simulink model "StopwatchSpec"  (R2017b)
settings: Solver=FixedStepDiscrete  StartTime=0.0  StopTime=20  FixedStep=1  RelTol=1e-3
model workspace (MAT data in the model file):
  ContractValidatorBlocksMap = containers.Map
  ContractValidatorBlocksMap.serialization.keys = {'StopwatchSpec/contract/validator'}
  ContractValidatorBlocksMap.serialization.values{1}.block = 'StopwatchSpec/contract/validator'
  ContractValidatorBlocksMap.serialization.values{1}.assumePorts = 1
  ContractValidatorBlocksMap.serialization.values{1}.guaranteePorts = 3
  ContractValidatorBlocksMap.serialization.values{1}.modeBlocksPorts = 3
  ContractValidatorBlocksMap.serialization.values{1}.portHandles.Inport = [348.002807617 349.003417969 350.003173828 351.002075195 352.002319336 353.002319336 354.004394531]
  ContractValidatorBlocksMap.serialization.values{1}.portHandles.Outport = 355.00402832
  ContractValidatorBlocksMap.serialization.values{1}.portHandles.Enable = []
  ContractValidatorBlocksMap.serialization.values{1}.portHandles.Trigger = []
  ContractValidatorBlocksMap.serialization.values{1}.portHandles.State = []
  ContractValidatorBlocksMap.serialization.values{1}.portHandles.LConn = []
  ContractValidatorBlocksMap.serialization.values{1}.portHandles.RConn = []
  ContractValidatorBlocksMap.serialization.values{1}.portHandles.Ifaction = []
  ContractValidatorBlocksMap.serialization.values{1}.portHandles.Reset = []
  ContractValidatorBlocksMap.serialization.values{1}.portConnectivity(1).Type = '1'
  ContractValidatorBlocksMap.serialization.values{1}.portConnectivity(1).Position = [490 -60]
  ContractValidatorBlocksMap.serialization.values{1}.portConnectivity(1).SrcBlock = 14.0024414062
  ContractValidatorBlocksMap.serialization.values{1}.portConnectivity(1).SrcPort = 0
  ContractValidatorBlocksMap.serialization.values{1}.portConnectivity(1).DstBlock = []
  ContractValidatorBlocksMap.serialization.values{1}.portConnectivity(1).DstPort = []
  ContractValidatorBlocksMap.serialization.values{1}.portConnectivity(2).Type = '2'
  ContractValidatorBlocksMap.serialization.values{1}.portConnectivity(2).Position = [490 35]
  ContractValidatorBlocksMap.serialization.values{1}.portConnectivity(2).SrcBlock = 117.002685547
  ContractValidatorBlocksMap.serialization.values{1}.portConnectivity(2).SrcPort = 0
  ContractValidatorBlocksMap.serialization.values{1}.portConnectivity(2).DstBlock = []
  ContractValidatorBlocksMap.serialization.values{1}.portConnectivity(2).DstPort = []
  ContractValidatorBlocksMap.serialization.values{1}.portConnectivity(3).Type = '3'
  ContractValidatorBlocksMap.serialization.values{1}.portConnectivity(3).Position = [490 130]
  ContractValidatorBlocksMap.serialization.values{1}.portConnectivity(3).SrcBlock = 84.0024414062
  ContractValidatorBlocksMap.serialization.values{1}.portConnectivity(3).SrcPort = 0
  ContractValidatorBlocksMap.serialization.values{1}.portConnectivity(3).DstBlock = []
  ContractValidatorBlocksMap.serialization.values{1}.portConnectivity(3).DstPort = []
  ContractValidatorBlocksMap.serialization.values{1}.portConnectivity(4).Type = '4'
  ContractValidatorBlocksMap.serialization.values{1}.portConnectivity(4).Position = [490 225]
  ContractValidatorBlocksMap.serialization.values{1}.portConnectivity(4).SrcBlock = 111.003662109
  ContractValidatorBlocksMap.serialization.values{1}.portConnectivity(4).SrcPort = 0
  ContractValidatorBlocksMap.serialization.values{1}.portConnectivity(4).DstBlock = []
  ContractValidatorBlocksMap.serialization.values{1}.portConnectivity(4).DstPort = []
  ContractValidatorBlocksMap.serialization.values{1}.portConnectivity(5).Type = '5'
  ContractValidatorBlocksMap.serialization.values{1}.portConnectivity(5).Position = [490 320]
  ContractValidatorBlocksMap.serialization.values{1}.portConnectivity(5).SrcBlock = 175.004272461
  ContractValidatorBlocksMap.serialization.values{1}.portConnectivity(5).SrcPort = 0
  ContractValidatorBlocksMap.serialization.values{1}.portConnectivity(5).DstBlock = []
  ContractValidatorBlocksMap.serialization.values{1}.portConnectivity(5).DstPort = []
  ContractValidatorBlocksMap.serialization.values{1}.portConnectivity(6).Type = '6'
  ContractValidatorBlocksMap.serialization.values{1}.portConnectivity(6).Position = [490 415]
  ContractValidatorBlocksMap.serialization.values{1}.portConnectivity(6).SrcBlock = 186.00378418
  ContractValidatorBlocksMap.serialization.values{1}.portConnectivity(6).SrcPort = 0
  ContractValidatorBlocksMap.serialization.values{1}.portConnectivity(6).DstBlock = []
  ContractValidatorBlocksMap.serialization.values{1}.portConnectivity(6).DstPort = []
  ContractValidatorBlocksMap.serialization.values{1}.portConnectivity(7).Type = '7'
  ContractValidatorBlocksMap.serialization.values{1}.portConnectivity(7).Position = [490 510]
  ContractValidatorBlocksMap.serialization.values{1}.portConnectivity(7).SrcBlock = 197.002929688
  ContractValidatorBlocksMap.serialization.values{1}.portConnectivity(7).SrcPort = 0
  ContractValidatorBlocksMap.serialization.values{1}.portConnectivity(7).DstBlock = []
  ContractValidatorBlocksMap.serialization.values{1}.portConnectivity(7).DstPort = []
  ContractValidatorBlocksMap.serialization.values{1}.portConnectivity(8).Type = '1'
  ContractValidatorBlocksMap.serialization.values{1}.portConnectivity(8).Position = [595 225]
  ContractValidatorBlocksMap.serialization.values{1}.portConnectivity(8).SrcBlock = []
  ContractValidatorBlocksMap.serialization.values{1}.portConnectivity(8).SrcPort = []
  ContractValidatorBlocksMap.serialization.values{1}.portConnectivity(8).DstBlock = 209.004150391
  ContractValidatorBlocksMap.serialization.values{1}.portConnectivity(8).DstPort = 0
  ContractValidatorBlocksMap.serialization.uniformity = 0
  ContractValidatorBlocksMap.serialization.keyType = 'char'
  ContractValidatorBlocksMap.serialization.valueType = 'any'
undefined symbols (not defined in the file or in its folder): ArrowOperator, contractAfterSimulation, ContractAssumeBlock, contractBeforeSimulation, ContractBlock, ContractEnsureBlock, ContractGuaranteeBlock, ContractModeBlock, ContractRequireBlock, ContractValidatorBlock, saveValidatorParameters
libraries: simulink x7, Kind x1
settings Model: Creator=mahgoubyahia  LastModifiedBy=hbourbou
settings OptimizationCC: LifeSpan=inf
settings DebuggingCC: SFExecutionAtInitializationDiag=none
settings HardwareCC: ProdBitPerSizeT=32  ProdBitPerPtrDiffT=32  ProdWordSize=32  ProdHWDeviceType=Specified
settings CodeAppCC: StateflowObjectComments=on

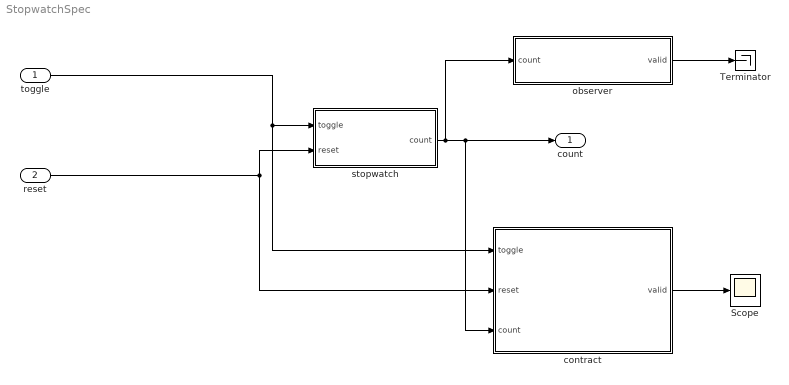
== system StopwatchSpec ==
  toggle : Inport
  reset : Inport  Port=2
  Scope : Scope
  Terminator : Terminator
  contract : Subsystem  AncestorBlock=Kind/contract  mask(ContractBlock){ContractBlockType=ContractBlock}
      mask DialogControl DescTextVar Prompt: Contract block
      mask Display:
      | text(0.5, 0.5, '{\bf\fontsize{20}Contract}', 'hor', 'center', 'texmode','on');
      | blocks = find_system(gcb, 'LookUnderMasks','all', 'SearchDepth',1,'BlockType','Inport');
      | for i = 1 : length(blocks)
      |     blockName = get_param(blocks(i), 'Name');
      |     [path, blockName] = fileparts(char(blockName));
      |     port_label('input', i, blockName);
      | end
      | 
      | blocks = find_system(gcb, 'LookUnderMasks','all', 'SearchDepth',1,'BlockType','Outport');
      | for i = 1 : length(blocks)
      |     blockName = get_param(blocks(i), 'Name');
      |     [path, blockName] = fileparts(char(blockName));
      |     port_label('output', i, blockName);
      | end
  observer : Subsystem  TreatAsAtomicUnit=on  mask(Observer){AnnotationType=ensures, ObserverType=ellipsoid}
      mask prompts: AnnotationType "Type of annotation (pre/post...)"; ObserverType "Observer type"
      mask help:
      | Set an observer for the system.
      | The annotation type parameter sets the type of observer:
      | - requires : pre-condition
      | - ensures : post-condition
      | - assert : an assertion
      | - observer : the observer computes a special type of properties
      mask TypeOptions AnnotationType: ensures | requires | assert | observer
      mask Callback AnnotationType:
      | paramStr = get_param(gcb, 'MaskValues');
      | 
      | if strcmp(paramStr{1}(1),'o')
      |     set_param(gcb,'MaskVisibilities',{'on';'on'});
      |     paramStr{2} = 'ellipsoid';
      |     set_param(gcb,'MaskValues',paramStr);
      | else
      |     set_param(gcb,'MaskVisibilities',{'on';'off'});
      | end
      mask Callback ObserverType:
      | paramStr = get_param(gcb, 'MaskValues');
      | 
      | if strcmp(paramStr{1}(1),'observer')
      |     set_param(gcb,'MaskVisibilities',{'on';'on'});
      |     paramStr{2} = 'ellipsoid';
      |     set_param(gcb,'MaskValues',paramStr);
      | else
      |     set_param(gcb,'MaskVisibilities',{'on';'off'});
      | end
      mask Display:
      | color('black');
      | text(0.5, 0.5, 'Observer Block', 'horizontalAlignment', 'center');
  stopwatch : Subsystem
  count : Outport
  wires:
  contract/1(valid) -> Scope/1
  reset/1 -> stopwatch/2(reset), contract/2(reset)
  toggle/1 -> contract/1(toggle), stopwatch/1(toggle)
  observer/1(valid) -> Terminator/1
  stopwatch/1(count) -> count/1, contract/3(count), observer/1(count)

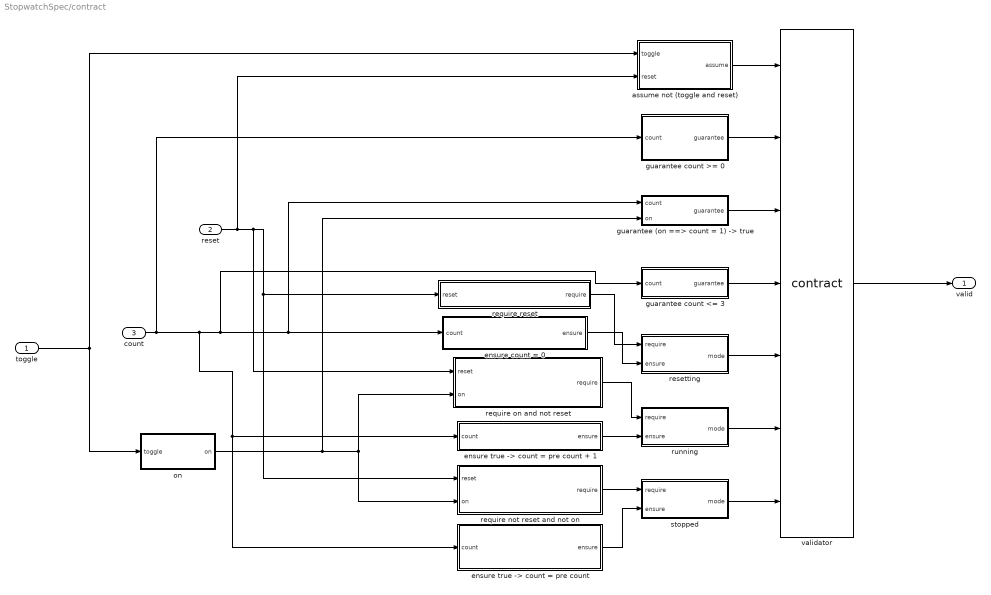
== system StopwatchSpec/contract ==
  toggle : Inport
  reset : Inport  Port=2
  count : Inport  Port=3  OutDataTypeStr=int32
  assume not (toggle and reset) : Subsystem  AncestorBlock=Kind/assume  mask(ContractAssumeBlock){ContractBlockType=ContractAssumeBlock}
      mask DialogControl DescTextVar Prompt: Assume block
  ensure count = 0 : Subsystem  AncestorBlock=Kind/ensure  mask(ContractEnsureBlock){ContractBlockType=ContractEnsureBlock}
      mask DialogControl DescTextVar Prompt: Ensure block
  "ensure true -> count = pre count" : Subsystem  AncestorBlock=Kind/ensure  mask(ContractEnsureBlock){ContractBlockType=ContractEnsureBlock}
      mask DialogControl DescTextVar Prompt: Ensure block
  "ensure true -> count = pre count + 1" : Subsystem  AncestorBlock=Kind/ensure  mask(ContractEnsureBlock){ContractBlockType=ContractEnsureBlock}
      mask DialogControl DescTextVar Prompt: Ensure block
  "guarantee (on ==> count = 1) -> true " : Subsystem  mask(ContractGuaranteeBlock){ContractBlockType=ContractGuaranteeBlock}
      mask DialogControl DescTextVar Prompt: Guarantee block
  guarantee count <= 3 : Subsystem  mask(ContractGuaranteeBlock){ContractBlockType=ContractGuaranteeBlock}
      mask DialogControl DescTextVar Prompt: Guarantee block
  guarantee count >= 0 : Subsystem  AncestorBlock=Kind/guarantee  mask(ContractGuaranteeBlock){ContractBlockType=ContractGuaranteeBlock}
      mask DialogControl DescTextVar Prompt: Guarantee block
  on : Subsystem
  require not reset and not on : Subsystem  AncestorBlock=Kind/require  mask(ContractRequireBlock){ContractBlockType=ContractRequireBlock}
      mask DialogControl DescTextVar Prompt: Require block
  require on and not reset : Subsystem  AncestorBlock=Kind/require  mask(ContractRequireBlock){ContractBlockType=ContractRequireBlock}
      mask DialogControl DescTextVar Prompt: Require block
  require reset : Subsystem  AncestorBlock=Kind/require  mask(ContractRequireBlock){ContractBlockType=ContractRequireBlock}
      mask DialogControl DescTextVar Prompt: Require block
  resetting : Subsystem  AncestorBlock=Kind/mode  mask(ContractModeBlock){ContractBlockType=ContractModeBlock}
      mask DialogControl DescTextVar Prompt: Mode block
  running : Subsystem  AncestorBlock=Kind/mode  mask(ContractModeBlock){ContractBlockType=ContractModeBlock}
      mask DialogControl DescTextVar Prompt: Mode block
  stopped : Subsystem  AncestorBlock=Kind/mode  mask(ContractModeBlock){ContractBlockType=ContractModeBlock}
      mask DialogControl DescTextVar Prompt: Mode block
  validator : M-S-Function  LoadFcn=saveValidatorParameters(gcb);  InitFcn=contractBeforeSimulation();  StopFcn=contractAfterSimulation();  FunctionName=contract  mask(ContractValidatorBlock){assumePorts=1, guaranteePorts=3, modePorts=3, ContractBlockType=ContractValidatorBlock, createInportsCheckbox=off}
      mask prompts: assumePorts "Assume ports     :"; guaranteePorts "Guarantee ports :"; modePorts "Mode ports        :"; createInportsCheckbox "Create inports and connect them automatically"
      mask init:
      | set_param(gcb,'LinkStatus','none');
      | contract_callback('inputs_callback',gcb);
      mask DialogControl DescTextVar Prompt: The validator block implements the following logic: <br> <br> <b>Sofar</b>(assume<sub>1</sub> <b>&#8743;</b> assume<sub>2</sub> <b>&#8743;</b> ... assume<sub>k</sub>) <b>&rarr;</b> (guarantee<sub>1</sub> <b>&#8743;</b> guarantee<sub>2</sub> <b>&#8743;</b> ... guarantee<sub>m</sub> <b>&#8743;</b>  mode<sub>1</sub> <b>&#8743;</b> mode<sub>2</sub> <b>&#8743;</b> ... <b>&#8743;</b> mode<sub>n</sub> )<br> where mode<sub>i</sub> = require<sub>i</sub> <b>&rarr;</b> ensure<sub>i</sub>
      mask Display:
      | color('black');
      | port_label('input',1,'assume');
      | port_label('input',2,'guarantee');
      | port_label('input',3,'guarantee');
      | port_label('input',4,'guarantee');
      | port_label('input',5,'mode');
      | port_label('input',6,'mode');
      | port_label('input',7,'mode');
      | port_label('output',1,'valid');
  valid : Outport
  wires:
  toggle/1 -> on/1(toggle), assume not (toggle and reset)/1(toggle)
  reset/1 -> require on and not reset/1(reset), require reset/1(reset), require not reset and not on/1(reset), assume not (toggle and reset)/2(reset)
  ensure count = 0/1(ensure) -> resetting/2(ensure)
  require on and not reset/1(require) -> running/1(require)
  "ensure true -> count = pre count + 1"/1(ensure) -> running/2(ensure)
  require not reset and not on/1(require) -> stopped/1(require)
  "ensure true -> count = pre count"/1(ensure) -> stopped/2(ensure)
  on/1(on) -> "guarantee (on ==> count = 1) -> true "/2(on), require on and not reset/2(on), require not reset and not on/2(on)
  count/1 -> guarantee count >= 0/1(count), "ensure true -> count = pre count"/1(count), "ensure true -> count = pre count + 1"/1(count), guarantee count <= 3/1(count), "guarantee (on ==> count = 1) -> true "/1(count), ensure count = 0/1(count)
  require reset/1(require) -> resetting/1(require)
  validator/1 -> valid/1
  assume not (toggle and reset)/1(assume) -> validator/1
  guarantee count >= 0/1(guarantee) -> validator/2
  "guarantee (on ==> count = 1) -> true "/1(guarantee) -> validator/3
  resetting/1(mode) -> validator/5
  running/1(mode) -> validator/6
  stopped/1(mode) -> validator/7
  guarantee count <= 3/1(guarantee) -> validator/4

== system StopwatchSpec/observer ==
  count : Inport
  Compare To Constant : simulink/Logic and Bit Operations/Compare To Constant  relop=<=  const=2  OutDataTypeStr=boolean
  valid : Outport
  wires:
  Compare To Constant/1 -> valid/1
  count/1 -> Compare To Constant/1

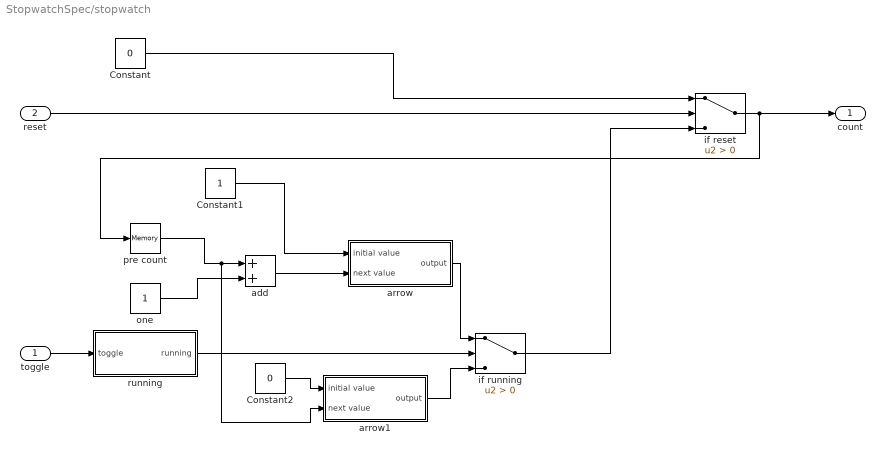
== system StopwatchSpec/stopwatch ==
  toggle : Inport
  reset : Inport  Port=2
  Constant : Constant  Value=0  OutDataTypeStr=int32
  Constant1 : Constant  OutDataTypeStr=int32
  Constant2 : Constant  Value=0  OutDataTypeStr=int32
  add : Sum
  arrow : Subsystem  mask{LustreOperatorBlock=ArrowOperator}
      mask prompts: LustreOperatorBlock "ArrowOperator"
  arrow1 : Subsystem  mask{LustreOperatorBlock=ArrowOperator}
      mask prompts: LustreOperatorBlock "ArrowOperator"
  if reset : Switch  Criteria=u2 > Threshold
  if running : Switch  Criteria=u2 > Threshold
  one : Constant  OutDataTypeStr=int32
  pre count : Memory
  running : Subsystem
  count : Outport
  wires:
  running/1(running) -> if running/2
  if reset/1 -> count/1, pre count/1
  if running/1 -> if reset/3
  reset/1 -> if reset/2
  Constant/1 -> if reset/1
  one/1 -> add/2
  toggle/1 -> running/1(toggle)
  Constant1/1 -> arrow/1(initial value)
  add/1 -> arrow/2(next value)
  arrow/1(output) -> if running/1
  pre count/1 -> arrow1/2(next value), add/1
  Constant2/1 -> arrow1/1(initial value)
  arrow1/1(output) -> if running/3

== system StopwatchSpec/contract/assume not (toggle and reset) ==
  toggle : Inport
  reset : Inport  Port=2
  and : Logic  IconShape=distinctive  AllPortsSameDT=off  OutDataTypeStr=boolean
  not : Logic  Operator=NOT  IconShape=distinctive  AllPortsSameDT=off  OutDataTypeStr=boolean
  assume : Outport  OutDataTypeStr=boolean
  wires:
  toggle/1 -> and/1
  reset/1 -> and/2
  and/1 -> not/1
  not/1 -> assume/1

== system StopwatchSpec/contract/ensure count = 0 ==
  count : Inport
  Compare To Zero : simulink/Logic and Bit Operations/Compare To Zero  relop===  OutDataTypeStr=boolean
  ensure : Outport  OutDataTypeStr=boolean
  wires:
  count/1 -> Compare To Zero/1
  Compare To Zero/1 -> ensure/1

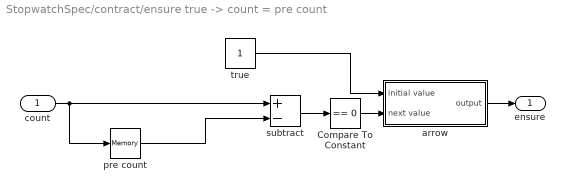
== system StopwatchSpec/contract/ensure true -> count = pre count ==
  count : Inport
  Compare To Constant : simulink/Logic and Bit Operations/Compare To Constant  relop===  const=0  OutDataTypeStr=boolean
  arrow : Subsystem  mask{LustreOperatorBlock=ArrowOperator}
      mask prompts: LustreOperatorBlock "ArrowOperator"
  pre count : Memory
  subtract : Sum  Inputs=+-
  true : Constant  OutDataTypeStr=boolean
  ensure : Outport  OutDataTypeStr=boolean
  wires:
  arrow/1(output) -> ensure/1
  pre count/1 -> subtract/2
  Compare To Constant/1 -> arrow/2(next value)
  count/1 -> pre count/1, subtract/1
  subtract/1 -> Compare To Constant/1
  true/1 -> arrow/1(initial value)

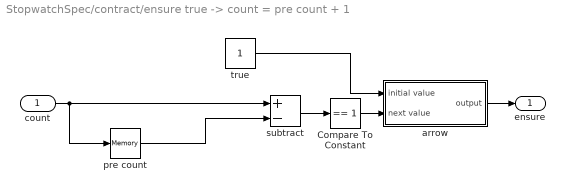
== system StopwatchSpec/contract/ensure true -> count = pre count + 1 ==
  count : Inport
  Compare To Constant : simulink/Logic and Bit Operations/Compare To Constant  relop===  const=1  OutDataTypeStr=boolean
  arrow : Subsystem  mask{LustreOperatorBlock=ArrowOperator}
      mask prompts: LustreOperatorBlock "ArrowOperator"
  pre count : Memory
  subtract : Sum  Inputs=+-
  true : Constant  OutDataTypeStr=boolean
  ensure : Outport  OutDataTypeStr=boolean
  wires:
  count/1 -> pre count/1, subtract/1
  subtract/1 -> Compare To Constant/1
  Compare To Constant/1 -> arrow/2(next value)
  true/1 -> arrow/1(initial value)
  arrow/1(output) -> ensure/1
  pre count/1 -> subtract/2

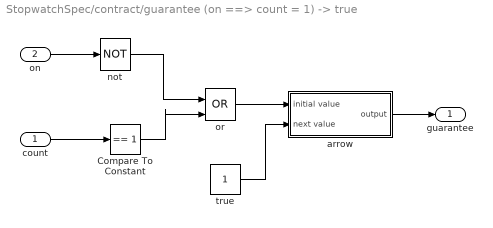
== system StopwatchSpec/contract/guarantee (on ==> count = 1) -> true  ==
  count : Inport  OutDataTypeStr=int32
  on : Inport  Port=2  OutDataTypeStr=boolean
  Compare To Constant : simulink/Logic and Bit Operations/Compare To Constant  relop===  const=1  OutDataTypeStr=boolean
  arrow : Subsystem  mask{LustreOperatorBlock=ArrowOperator}
      mask prompts: LustreOperatorBlock "ArrowOperator"
  not : Logic  Operator=NOT  IconShape=distinctive  AllPortsSameDT=off  OutDataTypeStr=boolean
  or : Logic  Operator=OR  IconShape=distinctive  AllPortsSameDT=off  OutDataTypeStr=boolean
  true : Constant  OutDataTypeStr=boolean
  guarantee : Outport  OutDataTypeStr=boolean
  wires:
  count/1 -> Compare To Constant/1
  Compare To Constant/1 -> or/2
  on/1 -> not/1
  not/1 -> or/1
  or/1 -> arrow/1(initial value)
  true/1 -> arrow/2(next value)
  arrow/1(output) -> guarantee/1

== system StopwatchSpec/contract/guarantee count <= 3 ==
  count : Inport
  Compare To Constant : simulink/Logic and Bit Operations/Compare To Constant  relop=<=  const=3.0  OutDataTypeStr=boolean
  guarantee : Outport  OutDataTypeStr=boolean
  wires:
  count/1 -> Compare To Constant/1
  Compare To Constant/1 -> guarantee/1

== system StopwatchSpec/contract/guarantee count >= 0 ==
  count : Inport
  Compare To Zero : simulink/Logic and Bit Operations/Compare To Zero  relop=>=  OutDataTypeStr=boolean
  guarantee : Outport  OutDataTypeStr=boolean
  wires:
  count/1 -> Compare To Zero/1
  Compare To Zero/1 -> guarantee/1

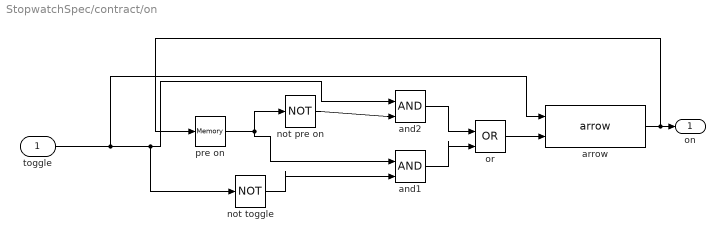
== system StopwatchSpec/contract/on ==
  toggle : Inport
  and1 : Logic  IconShape=distinctive  AllPortsSameDT=off  OutDataTypeStr=boolean
  and2 : Logic  IconShape=distinctive  AllPortsSameDT=off  OutDataTypeStr=boolean
  arrow : Kind/arrow  LustreOperatorBlock=ArrowOperator
  not pre on : Logic  Operator=NOT  IconShape=distinctive  AllPortsSameDT=off  OutDataTypeStr=boolean
  not toggle : Logic  Operator=NOT  IconShape=distinctive  AllPortsSameDT=off  OutDataTypeStr=boolean
  or : Logic  Operator=OR  IconShape=distinctive  AllPortsSameDT=off  OutDataTypeStr=boolean
  pre on : Memory
  on : Outport
  wires:
  toggle/1 -> arrow/1, not toggle/1, and2/1
  not toggle/1 -> and1/2
  pre on/1 -> and1/1, not pre on/1
  not pre on/1 -> and2/2
  and2/1 -> or/1
  and1/1 -> or/2
  or/1 -> arrow/2
  arrow/1 -> pre on/1, on/1

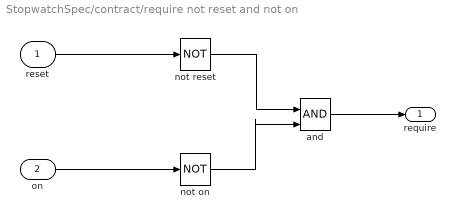
== system StopwatchSpec/contract/require not reset and not on ==
  reset : Inport
  on : Inport  Port=2
  and : Logic  IconShape=distinctive  AllPortsSameDT=off  OutDataTypeStr=boolean
  not on : Logic  Operator=NOT  IconShape=distinctive  AllPortsSameDT=off  OutDataTypeStr=boolean
  not reset : Logic  Operator=NOT  IconShape=distinctive  AllPortsSameDT=off  OutDataTypeStr=boolean
  require : Outport  OutDataTypeStr=boolean
  wires:
  reset/1 -> not reset/1
  on/1 -> not on/1
  not reset/1 -> and/1
  not on/1 -> and/2
  and/1 -> require/1

== system StopwatchSpec/contract/require on and not reset ==
  reset : Inport
  on : Inport  Port=2
  and : Logic  IconShape=distinctive  AllPortsSameDT=off  OutDataTypeStr=boolean
  not reset : Logic  Operator=NOT  IconShape=distinctive  AllPortsSameDT=off  OutDataTypeStr=boolean
  require : Outport  OutDataTypeStr=boolean
  wires:
  on/1 -> and/2
  reset/1 -> not reset/1
  not reset/1 -> and/1
  and/1 -> require/1

== system StopwatchSpec/contract/require reset ==
  reset : Inport
  require : Outport  OutDataTypeStr=boolean
  wires:
  reset/1 -> require/1

== system StopwatchSpec/contract/resetting ==
  note: Shouldn't not be edited
  require : Inport  OutDataTypeStr=boolean
  ensure : Inport  Port=2  OutDataTypeStr=boolean
  and : Logic  Operator=NOT  IconShape=distinctive  AllPortsSameDT=off  OutDataTypeStr=boolean
  or : Logic  Operator=OR  IconShape=distinctive  AllPortsSameDT=off  OutDataTypeStr=boolean
  mode : Outport
  wires:
  require/1 -> and/1
  ensure/1 -> or/2
  and/1 -> or/1
  or/1 -> mode/1

== system StopwatchSpec/contract/running ==
  note: Shouldn't not be edited
  require : Inport  OutDataTypeStr=boolean
  ensure : Inport  Port=2  OutDataTypeStr=boolean
  and : Logic  Operator=NOT  IconShape=distinctive  AllPortsSameDT=off  OutDataTypeStr=boolean
  or : Logic  Operator=OR  IconShape=distinctive  AllPortsSameDT=off  OutDataTypeStr=boolean
  mode : Outport
  wires:
  require/1 -> and/1
  ensure/1 -> or/2
  and/1 -> or/1
  or/1 -> mode/1

== system StopwatchSpec/contract/stopped ==
  note: Shouldn't not be edited
  require : Inport  OutDataTypeStr=boolean
  ensure : Inport  Port=2  OutDataTypeStr=boolean
  and : Logic  Operator=NOT  IconShape=distinctive  AllPortsSameDT=off  OutDataTypeStr=boolean
  or : Logic  Operator=OR  IconShape=distinctive  AllPortsSameDT=off  OutDataTypeStr=boolean
  mode : Outport
  wires:
  require/1 -> and/1
  ensure/1 -> or/2
  and/1 -> or/1
  or/1 -> mode/1

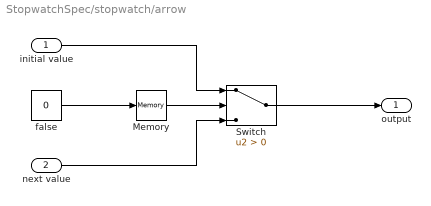
== system StopwatchSpec/stopwatch/arrow ==
  initial value : Inport
  next value : Inport  Port=2
  Memory : Memory  InitialCondition=1
  Switch : Switch  Criteria=u2 > Threshold
  false : Constant  Value=0  OutDataTypeStr=boolean
  output : Outport
  wires:
  Switch/1 -> output/1
  next value/1 -> Switch/3
  Memory/1 -> Switch/2
  false/1 -> Memory/1
  initial value/1 -> Switch/1

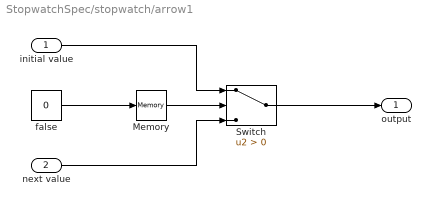
== system StopwatchSpec/stopwatch/arrow1 ==
  initial value : Inport
  next value : Inport  Port=2
  Memory : Memory  InitialCondition=1
  Switch : Switch  Criteria=u2 > Threshold
  false : Constant  Value=0  OutDataTypeStr=boolean
  output : Outport
  wires:
  Switch/1 -> output/1
  next value/1 -> Switch/3
  Memory/1 -> Switch/2
  false/1 -> Memory/1
  initial value/1 -> Switch/1

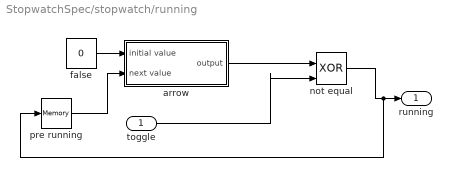
== system StopwatchSpec/stopwatch/running ==
  toggle : Inport
  arrow : Subsystem  mask{LustreOperatorBlock=ArrowOperator}
      mask prompts: LustreOperatorBlock "ArrowOperator"
  false : Constant  Value=0  OutDataTypeStr=boolean
  not equal : Logic  Operator=XOR  IconShape=distinctive  AllPortsSameDT=off  OutDataTypeStr=boolean
  pre running : Memory
  running : Outport
  wires:
  false/1 -> arrow/1(initial value)
  arrow/1(output) -> not equal/1
  not equal/1 -> pre running/1, running/1
  toggle/1 -> not equal/2
  pre running/1 -> arrow/2(next value)

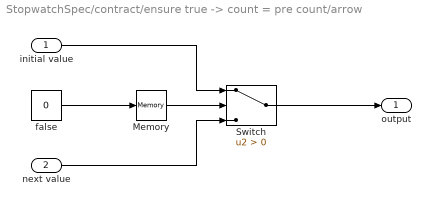
== system StopwatchSpec/contract/ensure true -> count = pre count/arrow ==
  initial value : Inport
  next value : Inport  Port=2
  Memory : Memory  InitialCondition=1
  Switch : Switch  Criteria=u2 > Threshold
  false : Constant  Value=0  OutDataTypeStr=boolean
  output : Outport
  wires:
  Switch/1 -> output/1
  next value/1 -> Switch/3
  Memory/1 -> Switch/2
  false/1 -> Memory/1
  initial value/1 -> Switch/1

== system StopwatchSpec/contract/ensure true -> count = pre count + 1/arrow ==
  initial value : Inport
  next value : Inport  Port=2
  Memory : Memory  InitialCondition=1
  Switch : Switch  Criteria=u2 > Threshold
  false : Constant  Value=0  OutDataTypeStr=boolean
  output : Outport
  wires:
  Switch/1 -> output/1
  next value/1 -> Switch/3
  Memory/1 -> Switch/2
  false/1 -> Memory/1
  initial value/1 -> Switch/1

== system StopwatchSpec/contract/guarantee (on ==> count = 1) -> true /arrow ==
  initial value : Inport
  next value : Inport  Port=2
  Memory : Memory  InitialCondition=1
  Switch : Switch  Criteria=u2 > Threshold
  false : Constant  Value=0  OutDataTypeStr=boolean
  output : Outport
  wires:
  Switch/1 -> output/1
  next value/1 -> Switch/3
  Memory/1 -> Switch/2
  false/1 -> Memory/1
  initial value/1 -> Switch/1

== system StopwatchSpec/stopwatch/running/arrow ==
  initial value : Inport
  next value : Inport  Port=2
  Memory : Memory  InitialCondition=1
  Switch : Switch  Criteria=u2 > Threshold
  false : Constant  Value=0  OutDataTypeStr=boolean
  output : Outport
  wires:
  Switch/1 -> output/1
  next value/1 -> Switch/3
  Memory/1 -> Switch/2
  false/1 -> Memory/1
  initial value/1 -> Switch/1
